simulink model "untitled"  (R2021b)
settings: Solver=VariableStepAuto  StartTime=0.0  StopTime=15  RelTol=1e-3
libraries: cstblocks x3
settings Model: Creator=lenovo  LastModifiedBy=lenovo

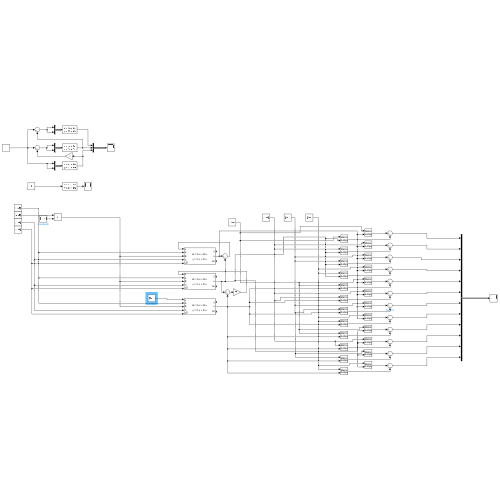
[thumbnail: Simulink's stored preview of the top-level diagram]
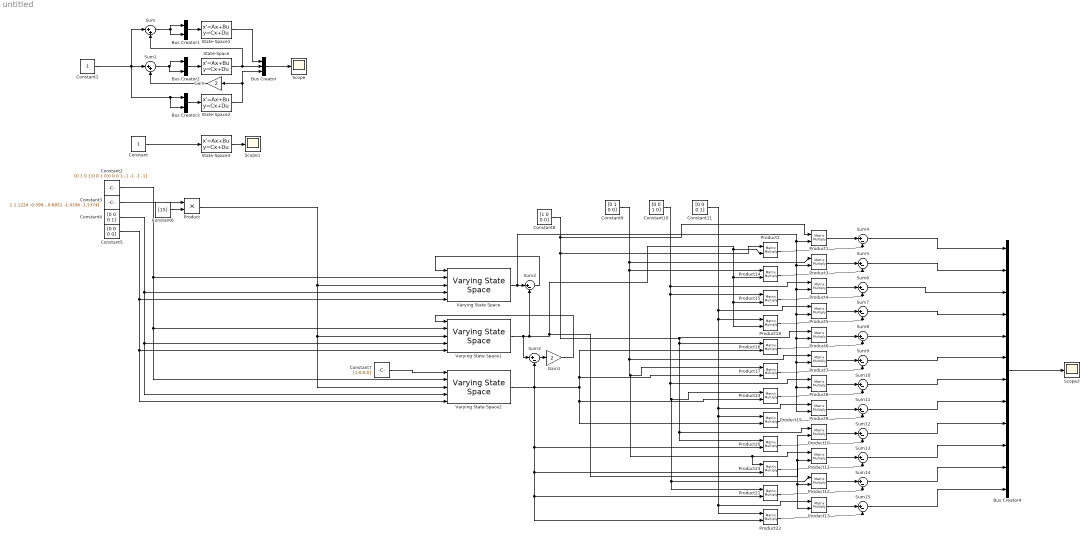
== system untitled ==
  Bus Creator : BusCreator  Inputs=3
  Bus Creator1 : BusCreator  Inputs=2
  Bus Creator2 : BusCreator  Inputs=2
  Bus Creator3 : BusCreator  Inputs=2
  Bus Creator4 : BusCreator  Inputs=12
  Constant : Constant
  Constant1 : Constant
  Constant10 : Constant  Value=[0 0 1 0]  VectorParams1D=off
  Constant11 : Constant  Value=[0 0 0 1]  VectorParams1D=off
  Constant2 : Constant  Value=[0 1 0 1;0 0 1 0;0 0 0 1;-1 -1 -1 -1]
  Constant3 : Constant  Value=[-1.1224 -0.5994 0.4404 0.1397;0 0 0 0;0 0 0 0;0.1397 -0.6851 -1.4336 -1.1374]
  Constant4 : Constant  Value=[0 0 0 1]  VectorParams1D=off
  Constant5 : Constant  Value=[0 0 0 0]  VectorParams1D=off
  Constant6 : Constant  Value=[15]  VectorParams1D=off
  Constant7 : Constant  Value=[1;0;0;0]  VectorParams1D=off
  Constant8 : Constant  Value=[1 0 0 0]  VectorParams1D=off
  Constant9 : Constant  Value=[0 1 0 0]  VectorParams1D=off
  Gain : Gain  Gain=2
  Gain1 : Gain  Gain=2
  Product : Product
  Product{1..24} (24 alike) : Product  Multiplication=Matrix(*)
  Scope : Scope
  Scope1 : Scope
  Scope2 : Scope
  State-Space : StateSpace  A=[0 1 0 1;0 0 1 0;0 0 0 1;-1 -1 -1 -1]  B=[1 0;0 0;0 0;0 1]  C=[0 0 0 1]  D=[0 0]  InitialCondition=0
  State-Space1 : StateSpace  A=[0 1 0 1;0 0 1 0;0 0 0 1;-1 -1 -1 -1]  B=[1 0;0 0;0 0;0 1]  C=[0 0 0 1]  D=[0 0]  InitialCondition=0
  State-Space2 : StateSpace  A=[0 1 0 1;0 0 1 0;0 0 0 1;-1 -1 -1 -1]  B=[1 0;0 0;0 0;0 1]  C=[0 0 0 1]  D=[0 0]  InitialCondition=0
  State-Space3 : StateSpace  A=[0 1 0 1;0 0 1 0;0 0 0 1;-1 -1 -1 -1]  B=[1;0;0;0]  C=[0 0 0 1]  D=[0]  InitialCondition=0
  Sum : Sum  Inputs=|++
  Sum1 : Sum  Inputs=|++
  Sum{2..15} (14 alike) : Sum  Inputs=|+-
  Varying State Space : cstblocks/Linear Parameter Varying/Varying State Space  x0=0  xNames=''  OutputX=on  OutputDX=on
  Varying State Space1 : cstblocks/Linear Parameter Varying/Varying State Space  x0=0  xNames=''  OutputX=on  OutputDX=on
  Varying State Space2 : cstblocks/Linear Parameter Varying/Varying State Space  x0=0  xNames=''  OutputX=on  OutputDX=on
  wires:
  State-Space/1 -> Bus Creator/2, Sum/2
  Constant1/1 -> Bus Creator3/2, Bus Creator3/1, Sum/1, Sum1/1
  State-Space2/1 -> Gain/1, Bus Creator/3
  Sum/1 -> Bus Creator1/2, Bus Creator1/1
  State-Space1/1 -> Bus Creator/1
  Sum1/1 -> Bus Creator2/2, Bus Creator2/1
  Gain/1 -> Sum1/2
  Bus Creator/1 -> Scope/1
  Bus Creator1/1 -> State-Space1/1
  Bus Creator2/1 -> State-Space/1
  Bus Creator3/1 -> State-Space2/1
  State-Space3/1 -> Scope1/1
  Constant/1 -> State-Space3/1
  Constant2/1 -> Varying State Space2/2, Varying State Space1/2, Varying State Space/2
  Constant4/1 -> Varying State Space2/4, Varying State Space1/4, Varying State Space/4
  Constant5/1 -> Varying State Space2/5, Varying State Space1/5, Varying State Space/5
  Constant7/1 -> Varying State Space2/1
  Bus Creator4/1 -> Scope2/1
  Varying State Space1/2 -> Product10/2, Product11/2, Product13/2, Product12/2, Product2/2, Product18/2, Product15/2, Product14/2, Sum2/2, Sum3/1
  Sum2/1 -> Varying State Space/1
  Sum3/1 -> Gain1/1
  Gain1/1 -> Varying State Space1/1
  Sum4/1 -> Bus Creator4/1
  Sum5/1 -> Bus Creator4/2
  Sum6/1 -> Bus Creator4/3
  Constant3/1 -> Product/1
  Constant6/1 -> Product/2
  Product/1 -> Varying State Space2/3, Varying State Space1/3, Varying State Space/3
  Sum7/1 -> Bus Creator4/4
  Sum8/1 -> Bus Creator4/5
  Sum9/1 -> Bus Creator4/6
  Sum10/1 -> Bus Creator4/7
  Sum11/1 -> Bus Creator4/8
  Sum12/1 -> Bus Creator4/9
  Sum13/1 -> Bus Creator4/10
  Sum14/1 -> Bus Creator4/11
  Sum15/1 -> Bus Creator4/12
  Constant8/1 -> Product1/1, Product2/1, Product20/1, Product10/1, Product16/1, Product6/1
  Product1/1 -> Sum4/1
  Product2/1 -> Sum4/2
  Product14/1 -> Sum5/2
  Product3/1 -> Sum5/1
  Product4/1 -> Sum6/1
  Product5/1 -> Sum7/1
  Product6/1 -> Sum8/1
  Product7/1 -> Sum9/1
  Product8/1 -> Sum10/1
  Product9/1 -> Sum11/1
  Product10/1 -> Sum12/1
  Product11/1 -> Sum13/1
  Product21/1 -> Sum14/2
  Product12/1 -> Sum14/1
  Product13/1 -> Sum15/1
  Product22/1 -> Sum15/2
  Product23/1 -> Sum13/2
  Product20/1 -> Sum12/2
  Product19/1 -> Sum11/2
  Product24/1 -> Sum10/2
  Product17/1 -> Sum9/2
  Product16/1 -> Sum8/2
  Product18/1 -> Sum7/2
  Product15/1 -> Sum6/2
  Constant9/1 -> Product3/1, Product17/1, Product11/1, Product23/1, Product7/1, Product14/1
  Constant11/1 -> Product22/1, Product13/1, Product19/1, Product9/1, Product18/1, Product5/1
  Constant10/1 -> Product21/1, Product12/1, Product24/1, Product8/1, Product15/1, Product4/1
  Varying State Space2/2 -> Product20/2, Product23/2, Product21/2, Product22/2, Sum3/2, Product19/2, Product24/2, Product17/2, Product16/2
  Varying State Space/2 -> Product1/2, Product9/2, Product8/2, Product7/2, Product6/2, Product5/2, Product4/2, Product3/2, Sum2/1
